simulink model "recentModel"  (R2020a)
settings: Solver=VariableStepAuto  StartTime=0.0  StopTime=15  RelTol=1e-3
undefined symbols (not defined in the file or in its folder): actors, ego, tracks
libraries: sim3dautolib x11, sim3dlib x1
settings Model: Creator=The MathWorks, Inc.  LastModifiedBy=Matze
settings DebuggingCC: SymbolicDimsDataTypeCodeGenerationDiagnostic=none

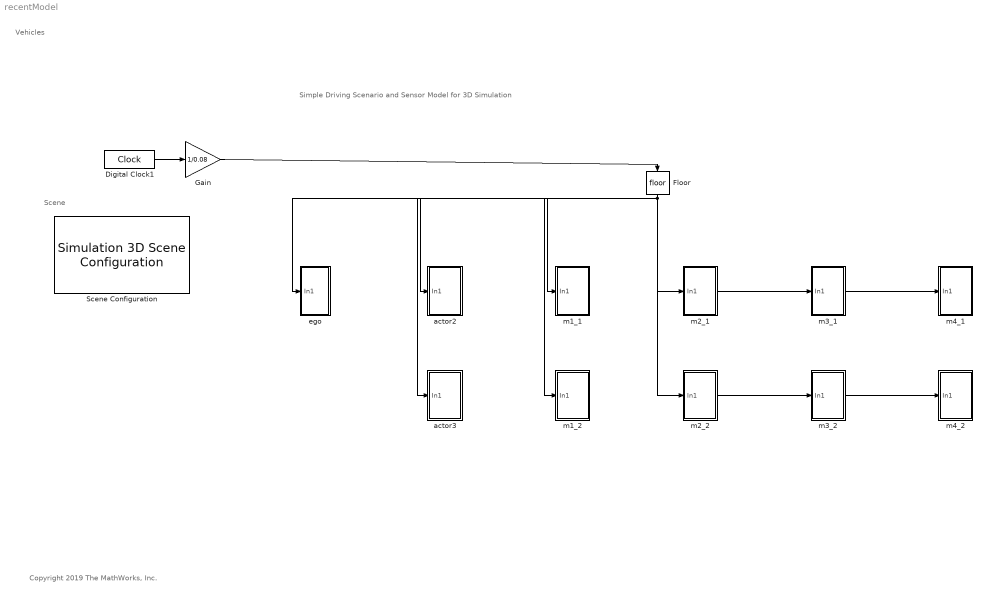
== system recentModel ==
  note: Vehicles
  note: Scene
  note: Copyright 2019 The MathWorks, Inc.
  note: Simple Driving Scenario and Sensor Model for 3D Simulation
  Digital Clock1 : DigitalClock  SampleTime=0.01
  Floor : Rounding
  Gain : Gain  Gain=1/0.08
  Scene Configuration : sim3dlib/Simulation 3D Scene Configuration  Priority=0  ProjectFormat=Default Scenes  SceneDesc=Straight road  ProjectName=VehicleSimulation.exe  ScenePath=/Game/Maps/HwStrght  vehTagList={'Actor2';'Actor3';'Scene Origin';'egoVehicle';'m1_1';'m1_2';'m2_1';'m2_2';'m3_1';'m3_2';'m4_1';'m4_2'}  vehTag=Actor2  OpVisEn=off  Ts=1/60  EnableWindow=on  sensorTag=MainCamera2  sensorId=2  sensorName=MainCamera2  mountLoc=Origin  offsetFlag=off  tmountOffset=[0, 0, 0]  rmountOffset=[0, 0, 0]  HorizontalResolution=1280  VerticalResolution=720  HorizontalFOV=60  mountPoint=[0 0 0]  mountOrientation=[0 0 0]  aMode=3  ID=2
      settings: SourceProductBaseCode=DR,VE
  actor2 : Subsystem
  actor3 : Subsystem
  ego : Subsystem
  m1_1 : Subsystem
  m1_2 : Subsystem
  m2_1 : Subsystem
  m2_2 : Subsystem
  m3_1 : Subsystem
  m3_2 : Subsystem
  m4_1 : Subsystem
  m4_2 : Subsystem
  wires:
  Gain/1 -> Floor/1
  Digital Clock1/1 -> Gain/1
  Floor/1 -> ego/1(In1), actor2/1(In1), actor3/1(In1), m1_1/1(In1), m1_2/1(In1), m2_1/1(In1), m2_2/1(In1), m3_1/1(In1), m3_2/1(In1), m4_1/1(In1), m4_2/1(In1)

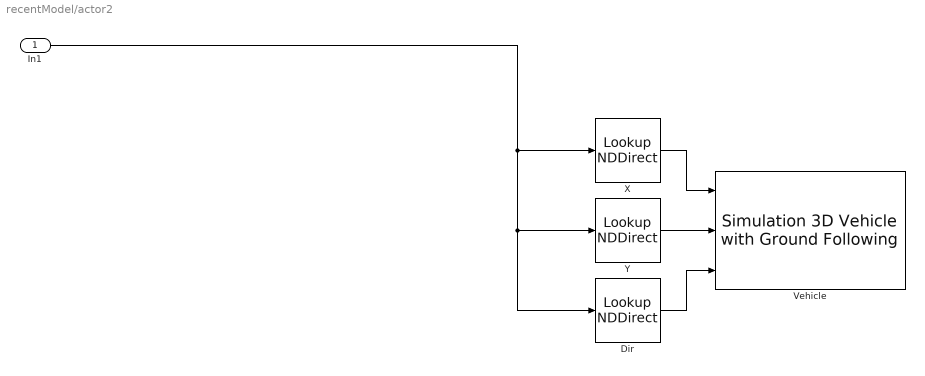
== system recentModel/actor2 ==
  In1 : Inport
  Dir : LookupNDDirect  NumberOfTableDimensions=1  Table=actors(2).dir
  Vehicle : sim3dautolib/Simulation 3D Vehicle with Ground Following  Priority=-1  PassVehMesh=Sport utility vehicle  VehColor=Green  InitialPos=[45, 10, 0]  InitialRot=[0, 0, 90]  ActorName=Actor2  SampleTime=-1  ActorType=SimulinkVehicle  ID=C  aMode=3  ActorTag=Actor2  CoordinateScheme=ISO  TransformOutportEnabled=off
      settings: SourceProductBaseCode=DR,VE
  X : LookupNDDirect  NumberOfTableDimensions=1  Table=actors(2).x
  Y : LookupNDDirect  NumberOfTableDimensions=1  Table=actors(2).y
  wires:
  Dir/1 -> Vehicle/3
  Y/1 -> Vehicle/2
  In1/1 -> X/1, Y/1, Dir/1
  X/1 -> Vehicle/1

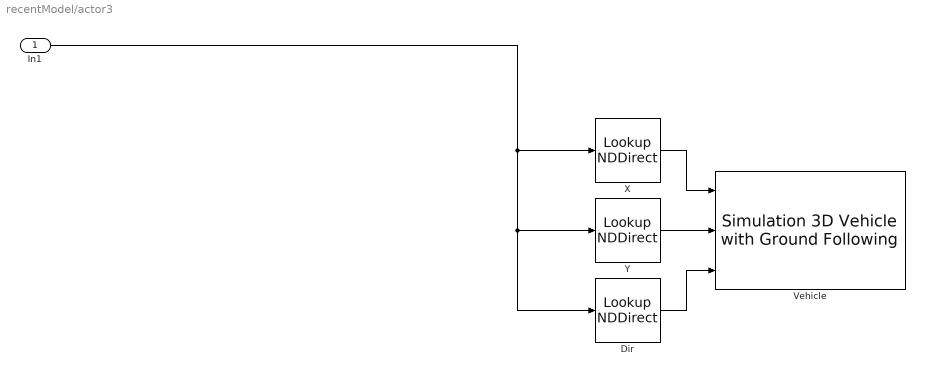
== system recentModel/actor3 ==
  In1 : Inport
  Dir : LookupNDDirect  NumberOfTableDimensions=1  Table=actors(3).dir
  Vehicle : sim3dautolib/Simulation 3D Vehicle with Ground Following  Priority=-1  PassVehMesh=Sport utility vehicle  VehColor=Green  InitialPos=[45, 10, 0]  InitialRot=[0, 0, 90]  ActorName=Actor3  SampleTime=-1  ActorType=SimulinkVehicle  ID=C  aMode=3  ActorTag=Actor3  CoordinateScheme=ISO  TransformOutportEnabled=off
      settings: SourceProductBaseCode=DR,VE
  X : LookupNDDirect  NumberOfTableDimensions=1  Table=actors(3).x
  Y : LookupNDDirect  NumberOfTableDimensions=1  Table=actors(3).y
  wires:
  Dir/1 -> Vehicle/3
  Y/1 -> Vehicle/2
  In1/1 -> X/1, Y/1, Dir/1
  X/1 -> Vehicle/1

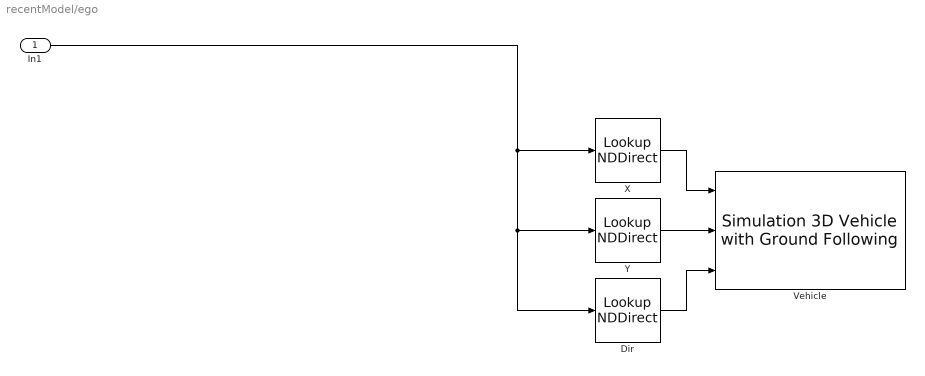
== system recentModel/ego ==
  In1 : Inport
  Dir : LookupNDDirect  NumberOfTableDimensions=1  Table=ego.dir
  Vehicle : sim3dautolib/Simulation 3D Vehicle with Ground Following  Priority=-1  PassVehMesh=Sport utility vehicle  VehColor=Red  InitialPos=[45, 10, 0]  InitialRot=[0, 0, 90]  ActorName=egoVehicle  SampleTime=-1  ActorType=SimulinkVehicle  ID=C  aMode=3  ActorTag=egoVehicle  CoordinateScheme=ISO  TransformOutportEnabled=off
      settings: SourceProductBaseCode=DR,VE
  X : LookupNDDirect  NumberOfTableDimensions=1  Table=ego.x
  Y : LookupNDDirect  NumberOfTableDimensions=1  Table=ego.y
  wires:
  Dir/1 -> Vehicle/3
  Y/1 -> Vehicle/2
  In1/1 -> X/1, Y/1, Dir/1
  X/1 -> Vehicle/1

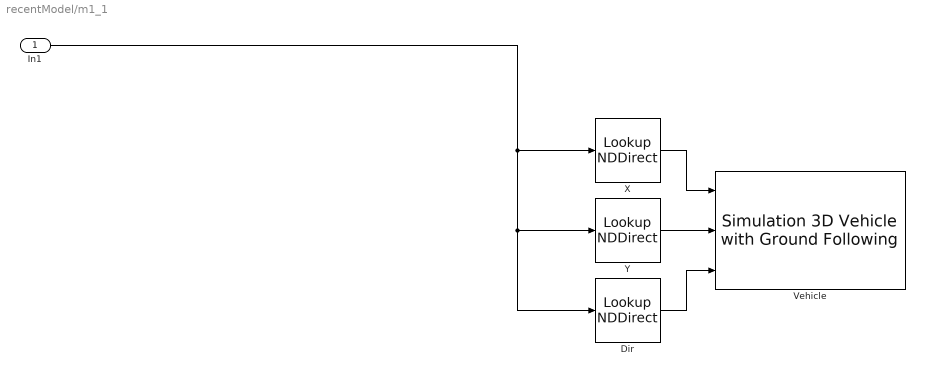
== system recentModel/m1_1 ==
  In1 : Inport
  Dir : LookupNDDirect  NumberOfTableDimensions=1  Table=tracks.m1(1).dir
  Vehicle : sim3dautolib/Simulation 3D Vehicle with Ground Following  Priority=-1  PassVehMesh=Sport utility vehicle  VehColor=Blue  InitialPos=[45, 10, 0]  InitialRot=[0, 0, 90]  ActorName=m1_1  SampleTime=-1  ActorType=SimulinkVehicle  ID=C  aMode=3  ActorTag=m1_1  CoordinateScheme=ISO  TransformOutportEnabled=off
      settings: SourceProductBaseCode=DR,VE
  X : LookupNDDirect  NumberOfTableDimensions=1  Table=tracks.m1(1).x
  Y : LookupNDDirect  NumberOfTableDimensions=1  Table=tracks.m1(1).y
  wires:
  Dir/1 -> Vehicle/3
  Y/1 -> Vehicle/2
  In1/1 -> X/1, Y/1, Dir/1
  X/1 -> Vehicle/1

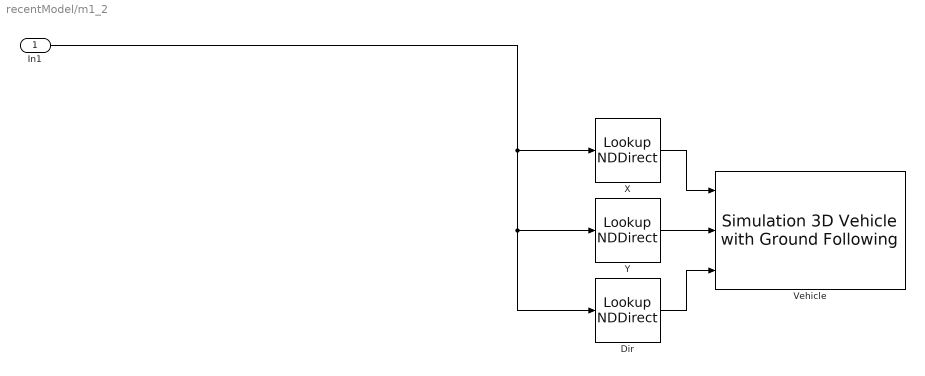
== system recentModel/m1_2 ==
  In1 : Inport
  Dir : LookupNDDirect  NumberOfTableDimensions=1  Table=tracks.m1(2).dir
  Vehicle : sim3dautolib/Simulation 3D Vehicle with Ground Following  Priority=-1  PassVehMesh=Sport utility vehicle  VehColor=Blue  InitialPos=[45, 10, 0]  InitialRot=[0, 0, 90]  ActorName=m1_2  SampleTime=-1  ActorType=SimulinkVehicle  ID=C  aMode=3  ActorTag=m1_2  CoordinateScheme=ISO  TransformOutportEnabled=off
      settings: SourceProductBaseCode=DR,VE
  X : LookupNDDirect  NumberOfTableDimensions=1  Table=tracks.m1(2).x
  Y : LookupNDDirect  NumberOfTableDimensions=1  Table=tracks.m1(2).y
  wires:
  Dir/1 -> Vehicle/3
  Y/1 -> Vehicle/2
  In1/1 -> X/1, Y/1, Dir/1
  X/1 -> Vehicle/1

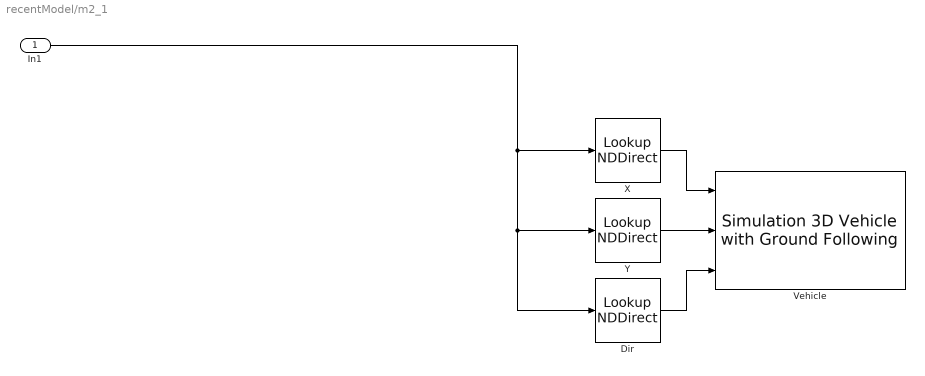
== system recentModel/m2_1 ==
  In1 : Inport
  Dir : LookupNDDirect  NumberOfTableDimensions=1  Table=tracks.m2(1).dir
  Vehicle : sim3dautolib/Simulation 3D Vehicle with Ground Following  Priority=-1  PassVehMesh=Sport utility vehicle  VehColor=Black  InitialPos=[45, 10, 0]  InitialRot=[0, 0, 90]  ActorName=m2_1  SampleTime=-1  ActorType=SimulinkVehicle  ID=C  aMode=3  ActorTag=m2_1  CoordinateScheme=ISO  TransformOutportEnabled=off
      settings: SourceProductBaseCode=DR,VE
  X : LookupNDDirect  NumberOfTableDimensions=1  Table=tracks.m2(1).x
  Y : LookupNDDirect  NumberOfTableDimensions=1  Table=tracks.m2(1).y
  wires:
  Dir/1 -> Vehicle/3
  Y/1 -> Vehicle/2
  In1/1 -> X/1, Y/1, Dir/1
  X/1 -> Vehicle/1

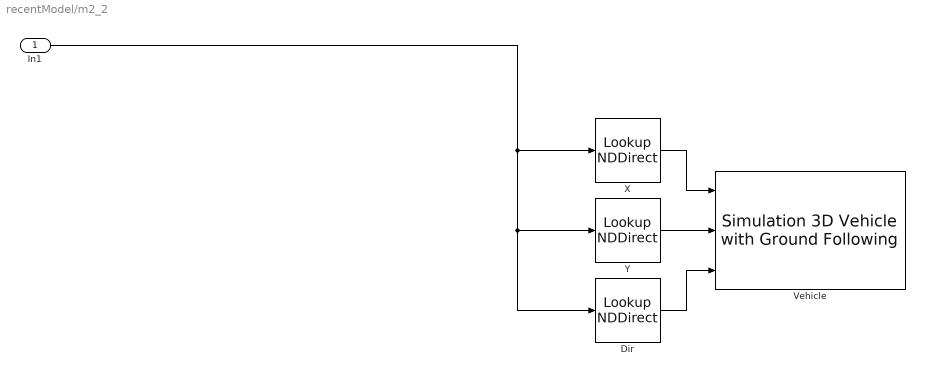
== system recentModel/m2_2 ==
  In1 : Inport
  Dir : LookupNDDirect  NumberOfTableDimensions=1  Table=tracks.m2(2).dir
  Vehicle : sim3dautolib/Simulation 3D Vehicle with Ground Following  Priority=-1  PassVehMesh=Sport utility vehicle  VehColor=Black  InitialPos=[45, 10, 0]  InitialRot=[0, 0, 90]  ActorName=m2_2  SampleTime=-1  ActorType=SimulinkVehicle  ID=C  aMode=3  ActorTag=m2_2  CoordinateScheme=ISO  TransformOutportEnabled=off
      settings: SourceProductBaseCode=DR,VE
  X : LookupNDDirect  NumberOfTableDimensions=1  Table=tracks.m2(2).x
  Y : LookupNDDirect  NumberOfTableDimensions=1  Table=tracks.m2(2).y
  wires:
  Dir/1 -> Vehicle/3
  Y/1 -> Vehicle/2
  In1/1 -> X/1, Y/1, Dir/1
  X/1 -> Vehicle/1

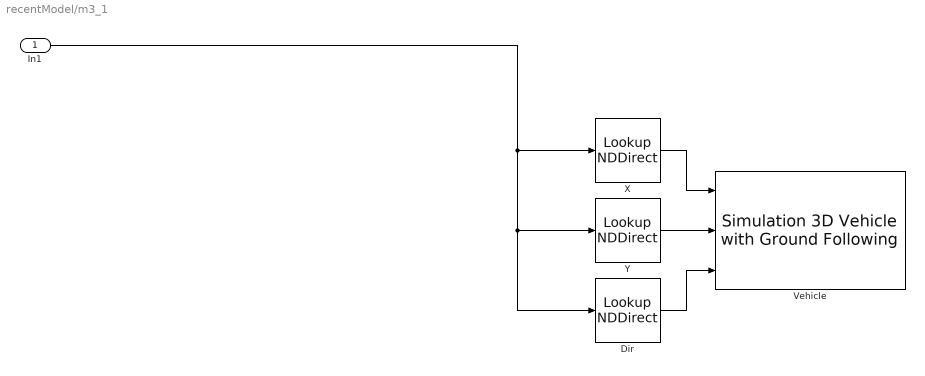
== system recentModel/m3_1 ==
  In1 : Inport
  Dir : LookupNDDirect  NumberOfTableDimensions=1  Table=tracks.m3(1).dir
  Vehicle : sim3dautolib/Simulation 3D Vehicle with Ground Following  Priority=-1  PassVehMesh=Sport utility vehicle  VehColor=Yellow  InitialPos=[45, 10, 0]  InitialRot=[0, 0, 90]  ActorName=m3_1  SampleTime=-1  ActorType=SimulinkVehicle  ID=C  aMode=3  ActorTag=m3_1  CoordinateScheme=ISO  TransformOutportEnabled=off
      settings: SourceProductBaseCode=DR,VE
  X : LookupNDDirect  NumberOfTableDimensions=1  Table=tracks.m3(1).x
  Y : LookupNDDirect  NumberOfTableDimensions=1  Table=tracks.m3(1).y
  wires:
  Dir/1 -> Vehicle/3
  Y/1 -> Vehicle/2
  In1/1 -> X/1, Y/1, Dir/1
  X/1 -> Vehicle/1

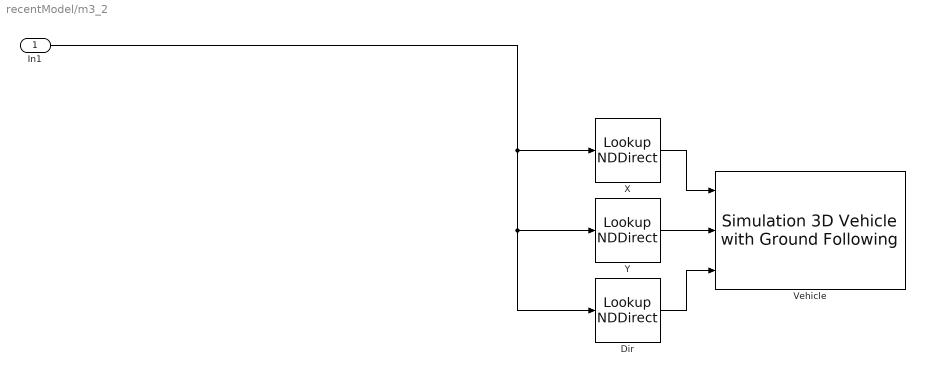
== system recentModel/m3_2 ==
  In1 : Inport
  Dir : LookupNDDirect  NumberOfTableDimensions=1  Table=tracks.m3(2).dir
  Vehicle : sim3dautolib/Simulation 3D Vehicle with Ground Following  Priority=-1  PassVehMesh=Sport utility vehicle  VehColor=Yellow  InitialPos=[45, 10, 0]  InitialRot=[0, 0, 90]  ActorName=m3_2  SampleTime=-1  ActorType=SimulinkVehicle  ID=C  aMode=3  ActorTag=m3_2  CoordinateScheme=ISO  TransformOutportEnabled=off
      settings: SourceProductBaseCode=DR,VE
  X : LookupNDDirect  NumberOfTableDimensions=1  Table=tracks.m3(2).x
  Y : LookupNDDirect  NumberOfTableDimensions=1  Table=tracks.m3(2).y
  wires:
  Dir/1 -> Vehicle/3
  Y/1 -> Vehicle/2
  In1/1 -> X/1, Y/1, Dir/1
  X/1 -> Vehicle/1

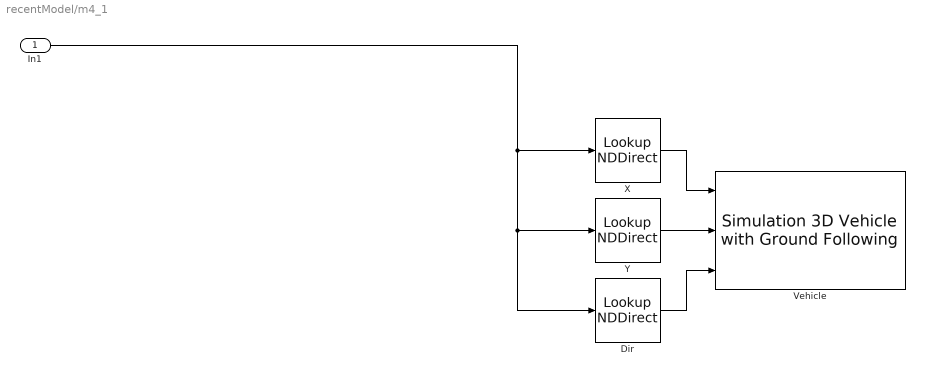
== system recentModel/m4_1 ==
  In1 : Inport
  Dir : LookupNDDirect  NumberOfTableDimensions=1  Table=tracks.m4(1).dir
  Vehicle : sim3dautolib/Simulation 3D Vehicle with Ground Following  Priority=-1  PassVehMesh=Sport utility vehicle  VehColor=Orange  InitialPos=[45, 10, 0]  InitialRot=[0, 0, 90]  ActorName=m4_1  SampleTime=-1  ActorType=SimulinkVehicle  ID=C  aMode=3  ActorTag=m4_1  CoordinateScheme=ISO  TransformOutportEnabled=off
      settings: SourceProductBaseCode=DR,VE
  X : LookupNDDirect  NumberOfTableDimensions=1  Table=tracks.m4(1).x
  Y : LookupNDDirect  NumberOfTableDimensions=1  Table=tracks.m4(1).y
  wires:
  Dir/1 -> Vehicle/3
  Y/1 -> Vehicle/2
  In1/1 -> X/1, Y/1, Dir/1
  X/1 -> Vehicle/1

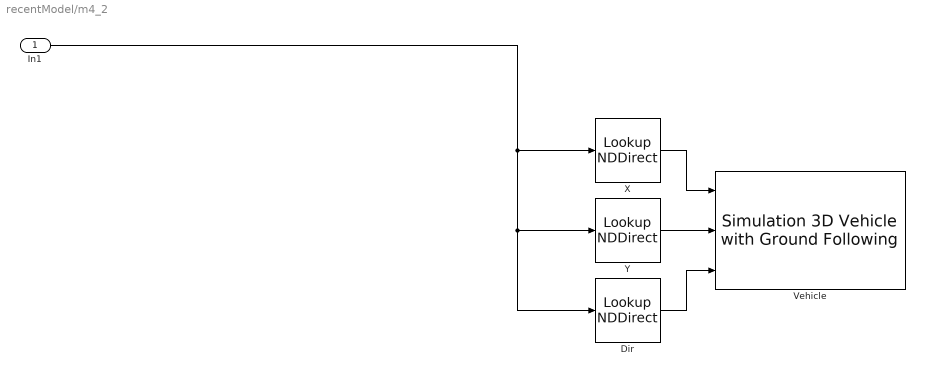
== system recentModel/m4_2 ==
  In1 : Inport
  Dir : LookupNDDirect  NumberOfTableDimensions=1  Table=tracks.m4(2).dir
  Vehicle : sim3dautolib/Simulation 3D Vehicle with Ground Following  Priority=-1  PassVehMesh=Sport utility vehicle  VehColor=Orange  InitialPos=[45, 10, 0]  InitialRot=[0, 0, 90]  ActorName=m4_2  SampleTime=-1  ActorType=SimulinkVehicle  ID=C  aMode=3  ActorTag=m4_2  CoordinateScheme=ISO  TransformOutportEnabled=off
      settings: SourceProductBaseCode=DR,VE
  X : LookupNDDirect  NumberOfTableDimensions=1  Table=tracks.m4(2).x
  Y : LookupNDDirect  NumberOfTableDimensions=1  Table=tracks.m4(2).y
  wires:
  Dir/1 -> Vehicle/3
  Y/1 -> Vehicle/2
  In1/1 -> X/1, Y/1, Dir/1
  X/1 -> Vehicle/1
